simulink model "s_reib1"  (Simulink 4.00)
settings: Solver=ode5  SolverMode=SingleTasking  StartTime=0.0  StopTime=50  FixedStep=0.1  MaxStep=0.1  RelTol=1e-3  AbsTol=1e-6
settings Model: LastModifiedBy=Administrator  Refine=4  SaveTime=off  SaveOutput=off  LimitDataPoints=off  BlockReductionOpt=off

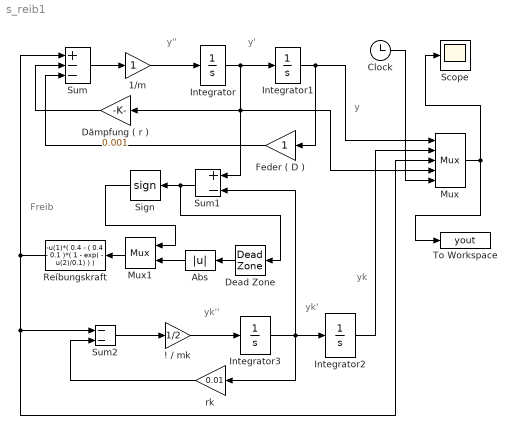
== system s_reib1 ==
  note: Freib
  note: yk
  note: y
  note: y''
  note: y'
  note: yk''
  note: yk'
  ! / mk : Gain  Gain=1/2  Multiplication=Element-wise(K.*u)  SaturateOnIntegerOverflow=on
  1/m : Gain  Gain=1  Multiplication=Element-wise(K.*u)  SaturateOnIntegerOverflow=on
  Abs : Abs  Orientation=left  SaturateOnIntegerOverflow=on
  Clock : Clock
      settings: DisplayTime=off  Decimation=10
  Dead Zone : DeadZone  Orientation=left  LowerValue=-0.01  UpperValue=0.01  SaturateOnIntegerOverflow=on  LinearizeAsGain=on
  Dämpfung ( r ) : Gain  Orientation=left  Gain=0.001  Multiplication=Element-wise(K.*u)  SaturateOnIntegerOverflow=on
  Feder ( D ) : Gain  Orientation=left  Gain=1  Multiplication=Element-wise(K.*u)  SaturateOnIntegerOverflow=on
  Integrator : Integrator  ExternalReset=none  InitialConditionSource=internal  InitialCondition=0  LimitOutput=off  UpperSaturationLimit=inf  LowerSaturationLimit=-inf  ShowSaturationPort=off  ShowStatePort=off  AbsoluteTolerance=auto
  Integrator1 : Integrator  ExternalReset=none  InitialConditionSource=internal  InitialCondition=2  LimitOutput=off  UpperSaturationLimit=inf  LowerSaturationLimit=-inf  ShowSaturationPort=off  ShowStatePort=off  AbsoluteTolerance=auto
  Integrator2 : Integrator  ExternalReset=none  InitialConditionSource=internal  InitialCondition=2  LimitOutput=off  UpperSaturationLimit=inf  LowerSaturationLimit=-inf  ShowSaturationPort=off  ShowStatePort=off  AbsoluteTolerance=auto
  Integrator3 : Integrator  ExternalReset=none  InitialConditionSource=internal  InitialCondition=0  LimitOutput=off  UpperSaturationLimit=inf  LowerSaturationLimit=-inf  ShowSaturationPort=off  ShowStatePort=off  AbsoluteTolerance=auto
  Mux : Mux  Inputs=5
      settings: DisplayOption=none
  Mux1 : Mux  Orientation=left  Inputs=2
      settings: DisplayOption=none
  Reíbungskraft : MATLABFcn  Orientation=left  MATLABFcn=-u(1)*( 0.4 - ( 0.4 - 0.1 )*( 1 - exp( - u(2)/0.1) ) )  OutputDimensions=1  OutputSignalType=auto  Output1D=on
  Scope : Scope
      settings: TickLabels=on  TimeRange=50  YMin=-2.5  YMax=22.5  SaveToWorkspace=off  SaveName=ScopeData  DataFormat=Array  LimitDataPoints=on  MaxDataPoints=5000
  Sign : Signum  Orientation=left
  Sum : Sum  Inputs=+--  SaturateOnIntegerOverflow=on
  Sum1 : Sum  Orientation=left  Inputs=+-  SaturateOnIntegerOverflow=on
  Sum2 : Sum  Inputs=--  SaturateOnIntegerOverflow=on
  To Workspace : ToWorkspace  VariableName=yout  SampleTime=0  SaveFormat=Array
      settings: MaxDataPoints=1000
  rk : Gain  Orientation=left  Gain=0.01  Multiplication=Element-wise(K.*u)  SaturateOnIntegerOverflow=on
  wires:
  Sum/1 -> 1/m/1
  1/m/1 -> Integrator/1
  Integrator/1 -> Integrator1/1, Dämpfung ( r )/1, Mux/4, Sum1/1
  Dämpfung ( r )/1 -> Sum/2
  Feder ( D )/1 -> Sum/3
  ! / mk/1 -> Integrator3/1
  Integrator1/1 -> Feder ( D )/1, Mux/1
  Integrator2/1 -> Mux/2
  Clock/1 -> Mux/5
  Reíbungskraft/1 -> Sum/1, Mux/3, Sum2/1
  Sum2/1 -> ! / mk/1
  Integrator3/1 -> Integrator2/1, Sum1/2, rk/1
  rk/1 -> Sum2/2
  Mux1/1 -> Reíbungskraft/1
  Sign/1 -> Mux1/1
  Sum1/1 -> Sign/1, Dead Zone/1
  Dead Zone/1 -> Abs/1
  Abs/1 -> Mux1/2
  Mux/1 -> To Workspace/1, Scope/1
